simulink library "lib_darwinop"  (R2013a)
settings: Solver=ode45  StartTime=0.0  StopTime=10.0  RelTol=1e-3
undefined symbols (not defined in the file or in its folder): darwinop_communication_setup
settings Model: Creator=florent  LastModifiedBy=florent

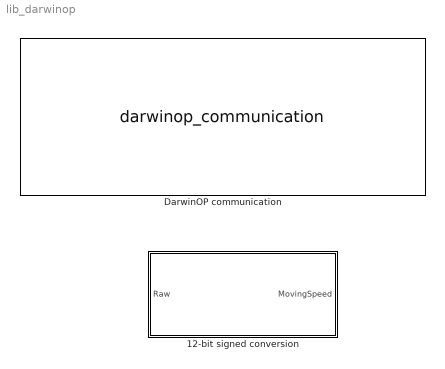
== system lib_darwinop ==
  12-bit signed conversion : MATLAB Function  TreatAsAtomicUnit=on
  DarwinOP communication : M-S-Function  StartFcn=darwinop_communication_setup('StartFcn');  StopFcn=darwinop_communication_setup('StopFcn');  FunctionName=darwinop_communication  Parameters=IP,Port,Protocol,SampleTime,Frame,ReadIndex,WriteIndex  mask{IP=192.168.123.1, Port=1234, Protocol=tcp, SampleTime=0.5, Frame=[ 2 1 36 6 3 1 30 2 0 0 2 200 44 6], ReadIndex=[ 1 2;3 2;5 2;7 2;9 2;11 2], WriteIndex=[ 9 2]}
      settings: DeleteFcn=darwinop_communication_setup('DeleteFcn');  ModelCloseFcn=darwinop_communication_setup('ModelCloseFcn');  NameChangeFcn=darwinop_communication_setup('NameChangeFcn');  OpenFcn=darwinop_communication_setup('OpenFcn');
      mask TypeOptions Protocol: tcp | udp
      mask Display:
      | image('darwin-blk.jpg')
      | 
      | port_label('output',1,'Right Shoulder Pitch(1)/Position')
      | port_label('output',2,'Right Shoulder Pitch(1)/Speed')
      | port_label('output',3,'Right Shoulder Pitch(1)/Load')
      | port_label('output',4,'Sub controller(200)/ACC X')
      | port_label('output',5,'Sub controller(200)/ACC Y')
      | port_label('output',6,'Sub controller(200)/ACC Z')
      | 
      | port_label('input',1,'Right Shoulder Pitch(1)/Goal Position')

== matlab function lib_darwinop/12-bit signed conversion ==
  data: Raw input; MovingSpeed output
function MovingSpeed = fcn(Raw)
%#codegen

Raw16 = uint16(Raw);
if bitand(Raw16,1024) ~= 0
    MovingSpeed = -double(bitand(Raw16,1023));
else
    MovingSpeed = double(bitand(Raw16,1023));
end
